simulink model "Clean_Tractor_Trailer_Flatness_v2"  (R2022b)
settings: Solver=ode4  StartTime=0.01  StopTime=20  FixedStep=0.01  RelTol=1e-3
InitFcn:
  | d0 = 1;
  | Dt=0.01;
  | 
  | %% if we want to "externalise" the trailer link from the car
  | a = 1.5;
  | 
  | %% distance between car and trailer
  | b = 2.5;
  | 
  | d1=b;
  | 
  | delay = 0.01;
  | 
  | %% delay with 0 signal before (to avoid instabilities before the "real" path following simulation")
  | del=2;
  | 
  | %% delay to sub above to chose starting using real value
  | dedel=1;
  | 
  | y0 = 0;
  | x0 = d1;
  | co=0;
  | 
  | the_pre=0;
  | the_pre_pre=0;
  | sdt=0.01;
  | 
  | ti_mod = 0.3;
  | 
  | phi0=pi;
  | 
  | %% Backward= pi, forward = 0
  | for_back=pi;
  | %%
  | 
  | %% Circle initial conditons forward
  | % for_back=0;
  | % dedel = 1.5;
  | % x_dot_init = 0;
  | % y_dot_init = 3;
  | % x_init = 0;
  | % y_init = 0;
  | % x0_init = b + del-dedel;
  | % y0_init = 0;
  | % theta0_init=for_back;
  | % theta1_init=0;
  | 
  | %% Circle initial conditons backward
  | % for_back=pi;
  | % dedel = 1.5;
  | % x_dot_init = 0;
  | % y_dot_init = 3;
  | % x_init = 0;
  | % y_init = 0;
  | % x0_init = -b;
  | % y0_init = 0;
  | % theta0_init=for_back;
  | % theta1_init=0;
  | 
  | %% func1 initial conditons
  | % x_dot_init = 1;
  | % y_dot_init = 0;
  | % x_init = 0;
  | % y_init = 0;
  | % x0_init = 0;
  | % y0_init = 0;
  | % theta0_init=0;
  | % theta1_init=0;
  | 
  | %% Wavy_up initial conditons
  | % x_dot_init = 0;
  | % y_dot_init = 0;
  | % x_init = 0;
  | % y_init = 0;
  | % x0_init = 0;
  | % y0_init = 0;
  | % theta0_init=0;
  | % theta1_init=0;
  | 
  | %% Backward Initial conditons for waving upward
  | for_back=pi;
  | x_dot_init = 1;
  | y_dot_init = 0;
  | 
  | x_init = 0;
  | y_init = 0;
  | 
  | %plant init
  | x0_init = -b;
  | y0_init = 0;
  | theta0_init=for_back;
  | theta1_init=0;
  | del=pi;
  | 
  | %% Forward Initial conditons for waving upward
  | % for_back=0;
  | % x_dot_init = 1;
  | % y_dot_init = 0;
  | %
  | % x_init = 0;
  | % y_init = 0;
  | %
  | % %plant init
  | % x0_init = b;
  | % y0_init = 0;
  | % theta0_init=for_back;
  | % theta1_init=0;
  | % del=pi;
  | 
  | 
  | %% Forward initial conditons for exp
  | % dedel=del;
  | % for_back=0;
  | % x_dot_init = 1;
  | % y_dot_init = 0;
  | % x_init = 0;
  | % y_init = 0;
  | % x0_init = 0;
  | % y0_init = 0;
  | % theta0_init=for_back;
  | % theta1_init=0;
  | 
  | %% Backward initial conditons for exp
  | % dedel=del-0.2;
  | % for_back=pi;
  | % x_dot_init = 1;
  | % y_dot_init = 0;
  | % x_init = 0;
  | % y_init = 0;
  | % x0_init = -b;
  | % y0_init = 0;
  | % theta0_init=for_back;
  | % theta1_init=0;
  | 
  | 
  | %% Cosinus initial conditons forward
  | % for_back=0;
  | % dedel=1;
  | % x_dot_init = 3;
  | % y_dot_init = 0;
  | % x_init = 0;
  | % y_init = 0;
  | % x0_init = b;
  | % y0_init = 0;
  | % theta0_init=for_back;
  | % theta1_init=0;
  | 
  | %% Cosinus initial conditons backward
  | % for_back=pi;
  | % dedel=1;
  | % x_dot_init = 3;
  | % y_dot_init = 0;
  | % x_init = 0;
  | % y_init = 0;
  | % x0_init = -b;
  | % y0_init = 0;
  | % theta0_init=for_back;
  | % theta1_init=0;
settings Model: Creator=chaudhuri  LastModifiedBy=Tugdual
settings ModelReferenceCC: EnableRefExpFcnMdlSchedulingChecks=on

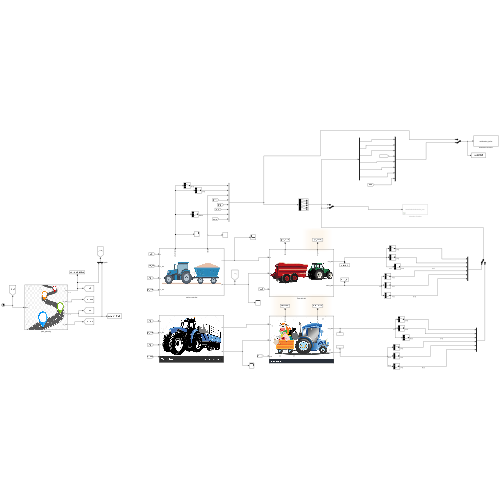
[thumbnail: Simulink's stored preview of the top-level diagram]
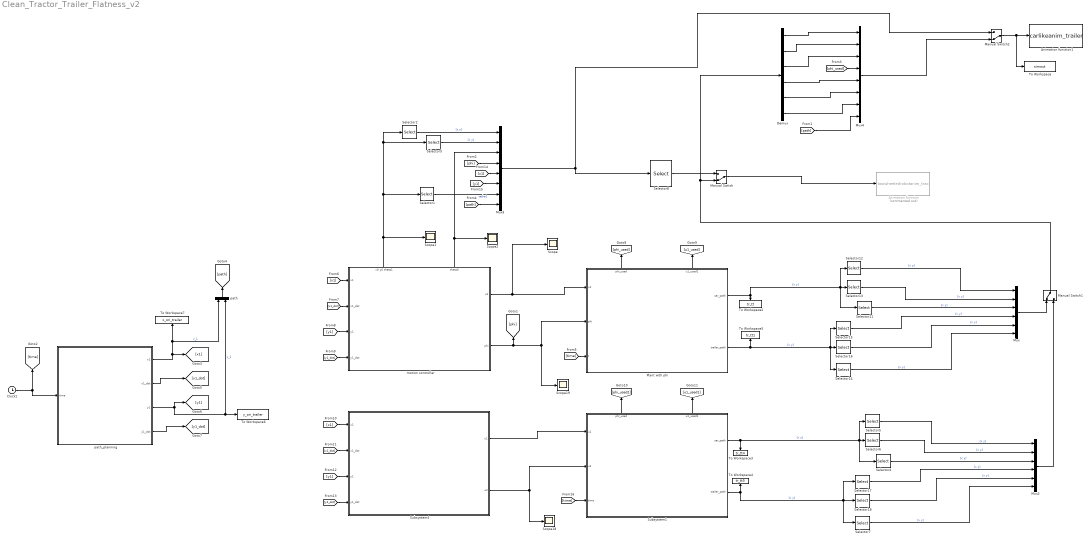
== system Clean_Tractor_Trailer_Flatness_v2 ==
  Animation function : S-Function  Commented=on  FunctionName=twowheeledrobotanim_trac  SFunctionDeploymentMode=off  EnableBusSupport=off
  Animation function1 : S-Function  FunctionName=carlikeanim_trailer  SFunctionDeploymentMode=off  EnableBusSupport=off
  Clock1 : Clock
  Demux : Demux  Outputs=6
  Manual Switch : ManualSwitch  CurrentSetting=0
  Manual Switch1 : ManualSwitch
  Manual Switch2 : ManualSwitch  CurrentSetting=0
  Mux : Mux  Inputs=6
  Mux2 : Mux  Inputs=6
  Mux3 : Mux  Inputs=8
  Mux4 : Mux  Inputs=8
  Plant with phi : Subsystem
      settings: PortSchema="{\"entries\":[{\"content\":{\"sides\":[{\"content\":{\"connectorIds\":[\"In1\",\"In2\",\"In3\"]},\"type\":\"ConnectorPlacement.EquallySpacedRectSide\",\"uuid\":\"e7db4861-1c7b-44d0-8ae0-043891a2d65e\"},{\"content\":{\"connectorIds\":[\"Out1\",\"Out2\"],\"side\":\"RIGHT\"},\"type\":\"ConnectorPlacement.EquallySpacedRectSide\",\"uuid\":\"ca6953ca-f3e9-441a-9b66-bf77f2babfba\"},{\"content\":{\"connectorIds\":[\"Out3\",\"Out4\"],\"side\":\"TOP\"},\"type\":\"ConnectorPlacement.EquallySpacedRectSide\",\"uuid\":\"0653e744-f46f-49ca-b3b7-6a2721aef055\"}]},\"type\":\"ConnectorPlacement.EquallySpacedConnector\",\"uuid\":\"d05efadf-1bd4-4ab0-9eff-99e9b7844dfa\"}],\"packageUris\":[\"http://schema.mathworks.com/mf0/Connector/R2020b\"],\"version\":\"1.0\"}"
      mask Display: image('$imagefile'); % Use "Edit Image" on toolstrip to change.
  Scope{,1..2,18..19} (5 alike) : Scope
  Selector{1,4,7,11,14} (5 alike) : Selector  InputPortWidth=3  IndexOptions=Index vector (dialog)  Indices=[3]  OutputSizes=1
  Selector{2,5,12,15,17} (5 alike) : Selector  InputPortWidth=3  IndexOptions=Index vector (dialog)  Indices=[1]  OutputSizes=1
  Selector{3,6,13,16,18} (5 alike) : Selector  InputPortWidth=3  IndexOptions=Index vector (dialog)  Indices=[2]  OutputSizes=1
  Selector8 : Selector  InputPortWidth=9  IndexOptions=Index vector (dialog)  Indices=[1 2 3 5 6 7]  OutputSizes=1
  Subsystem1 : Subsystem
      settings: PortSchema="{\"entries\":[{\"content\":{\"sides\":[{\"content\":{\"connectorIds\":[\"In1\",\"In2\",\"In3\"]},\"type\":\"ConnectorPlacement.EquallySpacedRectSide\",\"uuid\":\"e7db4861-1c7b-44d0-8ae0-043891a2d65e\"},{\"content\":{\"connectorIds\":[\"Out1\",\"Out2\"],\"side\":\"RIGHT\"},\"type\":\"ConnectorPlacement.EquallySpacedRectSide\",\"uuid\":\"ca6953ca-f3e9-441a-9b66-bf77f2babfba\"},{\"content\":{\"connectorIds\":[\"Out3\",\"Out4\"],\"side\":\"TOP\"},\"type\":\"ConnectorPlacement.EquallySpacedRectSide\",\"uuid\":\"0653e744-f46f-49ca-b3b7-6a2721aef055\"}]},\"type\":\"ConnectorPlacement.EquallySpacedConnector\",\"uuid\":\"d05efadf-1bd4-4ab0-9eff-99e9b7844dfa\"}],\"packageUris\":[\"http://schema.mathworks.com/mf0/Connector/R2020b\"],\"version\":\"1.0\"}"
      mask Display: image('$imagefile'); % Use "Edit Image" on toolstrip to change.
  Subsystem4 : Subsystem
      mask Display: image('$imagefile'); % Use "Edit Image" on toolstrip to change.
  To Workspace : ToWorkspace  VariableName=simout  SaveFormat=Timeseries  SampleTime=-1
  To Workspace2 : ToWorkspace  VariableName=tr_tt  SaveFormat=Timeseries  SampleTime=-1
  To Workspace3 : ToWorkspace  VariableName=tr_tt4  SaveFormat=Timeseries  SampleTime=-1
  To Workspace4 : ToWorkspace  VariableName=tr_tt5  SaveFormat=Timeseries  SampleTime=-1
  To Workspace5 : ToWorkspace  VariableName=tr_tt1  SaveFormat=Timeseries  SampleTime=-1
  To Workspace6 : ToWorkspace  VariableName=y_ori_trailer  SaveFormat=Timeseries  SampleTime=-1
      settings: Save2DSignal=2-D array (concatenate along first dimension)
  To Workspace7 : ToWorkspace  VariableName=x_ori_trailer  SaveFormat=Timeseries  SampleTime=-1
      settings: Save2DSignal=2-D array (concatenate along first dimension)
  motion controller : Subsystem
      settings: PortSchema="{\"entries\":[{\"content\":{\"sides\":[{\"content\":{\"connectorIds\":[\"In1\",\"In2\",\"In3\",\"In4\"]},\"type\":\"ConnectorPlacement.EquallySpacedRectSide\",\"uuid\":\"11bc3301-7ab6-4d38-8445-7de1e6050525\"},{\"content\":{\"connectorIds\":[\"Out1\",\"Out2\"],\"side\":\"RIGHT\"},\"type\":\"ConnectorPlacement.EquallySpacedRectSide\",\"uuid\":\"374bee85-8743-45f2-a60a-268bfdaad2ec\"},{\"content\":{\"connectorIds\":[\"Out3\",\"Out4\"],\"side\":\"TOP\"},\"type\":\"ConnectorPlacement.EquallySpacedRectSide\",\"uuid\":\"71c6a0a5-27e8-424b-8871-57b58ecd48a6\"}]},\"type\":\"ConnectorPlacement.EquallySpacedConnector\",\"uuid\":\"fb4e8639-9b4e-4508-bb82-15087a60f723\"}],\"packageUris\":[\"http://schema.mathworks.com/mf0/Connector/R2020b\"],\"version\":\"1.0\"}"
      mask Display: image('$imagefile'); % Use "Edit Image" on toolstrip to change.
  path : Mux  Inputs=2
  path_planning : Subsystem
      mask Display: image('$imagefile'); % Use "Edit Image" on toolstrip to change.
  wires:
  Subsystem4/1(u1) -> Subsystem1/1(u1)
  Subsystem4/2(u2) -> Scope18/1, Subsystem1/2(u2)
  Clock1/1 -> [time], path_planning/1(time)
  motion controller/2(phi) -> [phi], Plant with phi/2(phi), Scope19/1
  Plant with phi/1(car_path) -> Selector11/1, Selector12/1, Selector13/1, To Workspace2/1  "[x y]"
  Selector11/1 -> Mux/3  "[x y]"
  Selector12/1 -> Mux/1  "[x y]"
  Selector13/1 -> Mux/2  "[x y]"
  Selector16/1 -> Mux/5  "[x y]"
  Selector15/1 -> Mux/4  "[x y]"
  Plant with phi/2(trailer_path) -> Selector14/1, Selector15/1, Selector16/1, To Workspace5/1  "[x y]"
  Selector14/1 -> Mux/6  "[x y]"
  Manual Switch1/1 -> Demux/1, Manual Switch/2
  motion controller/1(u1) -> Plant with phi/1(u1), Scope/1
  motion controller/3(x0 y0 theta1) -> Scope1/1, Selector2/1, Selector3/1, Selector1/1
  Selector1/1 -> Mux3/7  "tetha1"
  Selector3/1 -> Mux3/2  "[x y]"
  Selector2/1 -> Mux3/1  "[x y]"
  Selector17/1 -> Mux2/4  "[x y]"
  Selector7/1 -> Mux2/6  "[x y]"
  Subsystem1/2(trailer_path) -> Selector7/1, Selector18/1, Selector17/1, To Workspace4/1  "[x y]"
  Selector18/1 -> Mux2/5  "[x y]"
  Subsystem1/1(car_path) -> Selector4/1, Selector5/1, Selector6/1, To Workspace3/1  "[x y]"
  Selector6/1 -> Mux2/2  "[x y]"
  Selector5/1 -> Mux2/1  "[x y]"
  Mux2/1 -> Manual Switch1/2
  Selector4/1 -> Mux2/3  "[x y]"
  Mux/1 -> Manual Switch1/1
  Manual Switch2/1 -> To Workspace/1, Animation function1/1
  Manual Switch/1 -> Animation function/1
  motion controller/4(theta0) -> Scope2/1, Mux3/3
  Mux4/1 -> Manual Switch2/2
  Mux3/1 -> Selector8/1, Manual Switch2/1
  Demux/1 -> Mux4/1
  Demux/2 -> Mux4/2
  Demux/3 -> Mux4/3
  Demux/4 -> Mux4/5
  Demux/5 -> Mux4/6
  Demux/6 -> Mux4/7
  path/1 -> [path]
  [path] -> Mux4/8
  [phi] -> Mux3/4
  [phi_used] -> Mux4/4
  [path] -> Mux3/8
  [time] -> Plant with phi/3(t)
  Selector8/1 -> Manual Switch/1
  [x1] -> Mux3/5
  [y1] -> Mux3/6
  [x1] -> motion controller/1(x1)
  [x1_dot] -> motion controller/2(x1_dot)
  [y1] -> motion controller/3(y1)
  [y1_dot] -> motion controller/4(y1_dot)
  [y1_dot] -> Subsystem4/4(y1_dot)
  [y1] -> Subsystem4/3(y1)
  [x1_dot] -> Subsystem4/2(x1_dot)
  [x1] -> Subsystem4/1(x1)
  path_planning/4(y1_dot) -> [y1_dot]
  path_planning/3(y1) -> [y1], To Workspace6/1, path/2  "y_1"
  path_planning/2(x1_dot) -> [x1_dot]
  path_planning/1(x1) -> path/1, To Workspace7/1, [x1]  "x_1"
  Plant with phi/3(phi_used) -> [phi_used]
  Plant with phi/4(u1_used1) -> [u1_used]
  [time] -> Subsystem1/3(time)
  Subsystem1/4(u1_used1) -> [u1_used1]
  Subsystem1/3(phi_used) -> [phi_used2]

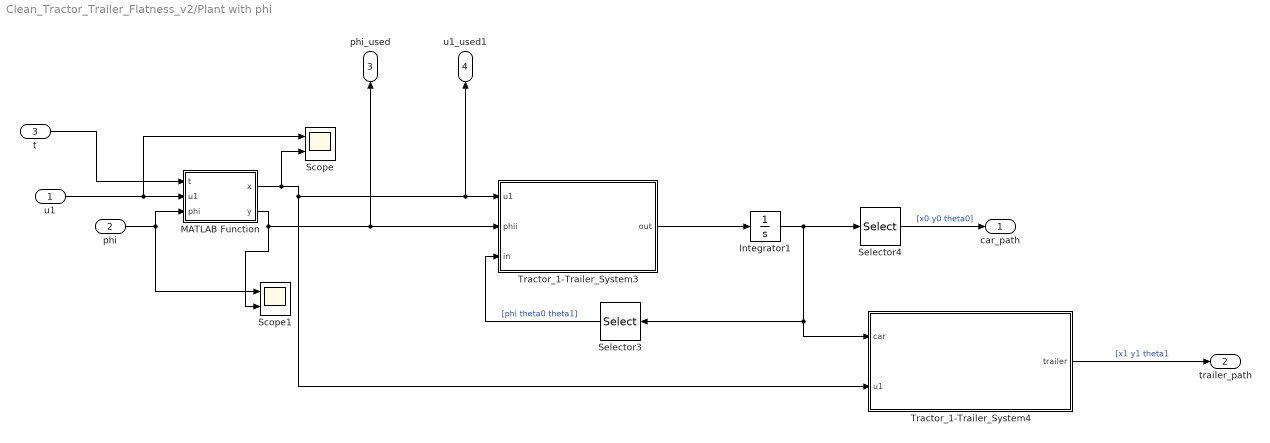
== system Clean_Tractor_Trailer_Flatness_v2/Plant with phi ==
  u1 : Inport
  phi : Inport  Port=2
  t : Inport  Port=3
  Integrator1 : Integrator  InitialCondition=[x0_init;y0_init;theta0_init;theta1_init]
  MATLAB Function : MATLAB Function  TreatAsAtomicUnit=on
  Scope : Scope  NumInputPorts=2
  Scope1 : Scope  NumInputPorts=2
  Selector3 : Selector  InputPortWidth=4  IndexOptions=Index vector (dialog)  Indices=[3 4]  OutputSizes=1
  Selector4 : Selector  InputPortWidth=4  IndexOptions=Index vector (dialog)  Indices=[1 2 3]  OutputSizes=1
  Tractor_1-Trailer_System3 : MATLAB Function  TreatAsAtomicUnit=on
  Tractor_1-Trailer_System4 : MATLAB Function  TreatAsAtomicUnit=on
  car_path : Outport
  trailer_path : Outport  Port=2
  phi_used : Outport  Port=3
  u1_used1 : Outport  Port=4
  wires:
  Tractor_1-Trailer_System4/1(trailer) -> trailer_path/1  "[x1 y1 theta1"
  Tractor_1-Trailer_System3/1(out) -> Integrator1/1
  Integrator1/1 -> Selector4/1, Tractor_1-Trailer_System4/1(car), Selector3/1
  Selector3/1 -> Tractor_1-Trailer_System3/3(in)  "[phi theta0 theta1]"
  Selector4/1 -> car_path/1  "[x0 y0 theta0]"
  MATLAB Function/2(y) -> Scope1/2, Tractor_1-Trailer_System3/2(phii), phi_used/1
  MATLAB Function/1(x) -> Scope/2, u1_used1/1, Tractor_1-Trailer_System3/1(u1), Tractor_1-Trailer_System4/2(u1)
  t/1 -> MATLAB Function/1(t)
  u1/1 -> Scope/1, MATLAB Function/2(u1)
  phi/1 -> Scope1/1, MATLAB Function/3(phi)

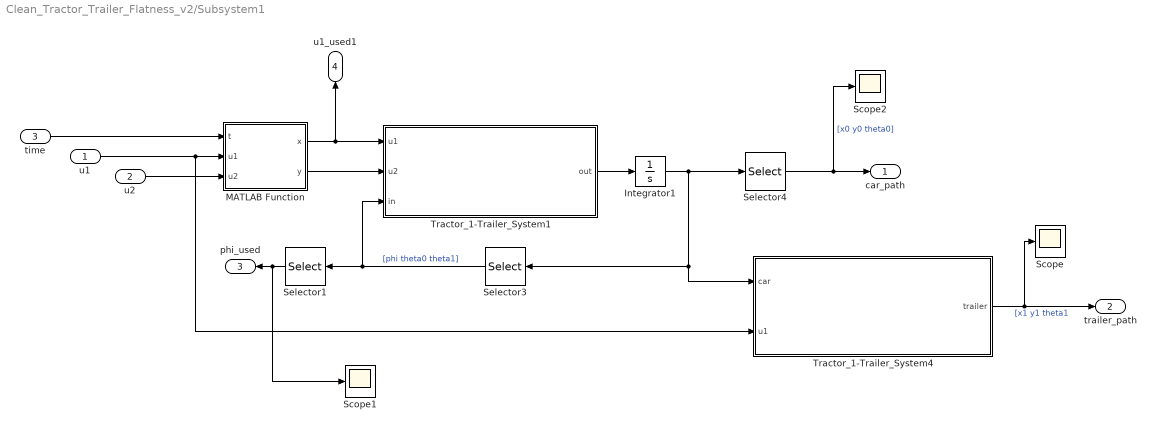
== system Clean_Tractor_Trailer_Flatness_v2/Subsystem1 ==
  u1 : Inport
  u2 : Inport  Port=2
  time : Inport  Port=3
  Integrator1 : Integrator  InitialCondition=[x0_init;y0_init;phi0;theta0_init;theta1_init]
  MATLAB Function : MATLAB Function  TreatAsAtomicUnit=on
  Scope : Scope
  Scope1 : Scope
  Scope2 : Scope
  Selector1 : Selector  InputPortWidth=3  IndexOptions=Index vector (dialog)  Indices=[1]  OutputSizes=1
  Selector3 : Selector  InputPortWidth=5  IndexOptions=Index vector (dialog)  Indices=[3 4 5]  OutputSizes=1
  Selector4 : Selector  InputPortWidth=5  IndexOptions=Index vector (dialog)  Indices=[1 2 4]  OutputSizes=1
  Tractor_1-Trailer_System1 : MATLAB Function  TreatAsAtomicUnit=on
  Tractor_1-Trailer_System4 : MATLAB Function  TreatAsAtomicUnit=on
  car_path : Outport
  trailer_path : Outport  Port=2
  phi_used : Outport  Port=3
  u1_used1 : Outport  Port=4
  wires:
  Tractor_1-Trailer_System4/1(trailer) -> Scope/1, trailer_path/1  "[x1 y1 theta1"
  Tractor_1-Trailer_System1/1(out) -> Integrator1/1
  Integrator1/1 -> Selector4/1, Tractor_1-Trailer_System4/1(car), Selector3/1
  Selector3/1 -> Selector1/1, Tractor_1-Trailer_System1/3(in)  "[phi theta0 theta1]"
  Selector4/1 -> Scope2/1, car_path/1  "[x0 y0 theta0]"
  u1/1 -> MATLAB Function/2(u1), Tractor_1-Trailer_System4/2(u1)
  u2/1 -> MATLAB Function/3(u2)
  time/1 -> MATLAB Function/1(t)
  MATLAB Function/1(x) -> u1_used1/1, Tractor_1-Trailer_System1/1(u1)
  MATLAB Function/2(y) -> Tractor_1-Trailer_System1/2(u2)
  Selector1/1 -> Scope1/1, phi_used/1

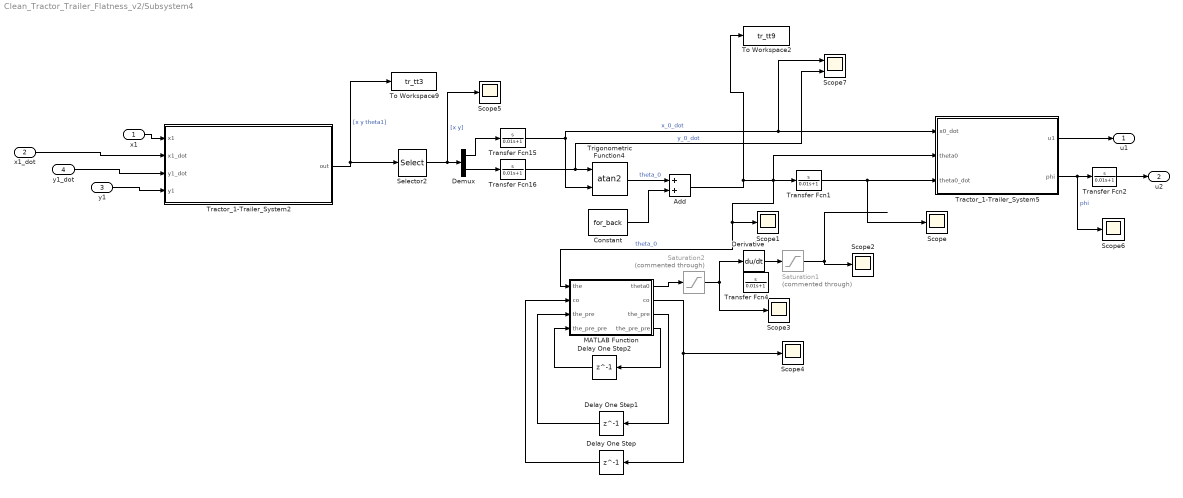
== system Clean_Tractor_Trailer_Flatness_v2/Subsystem4 ==
  x1 : Inport
  x1_dot : Inport  Port=2
  y1 : Inport  Port=3
  y1_dot : Inport  Port=4
  Add : Sum
  Constant : Constant  Value=for_back
  Delay One Step : Delay  DelayLength=1
  Delay One Step1 : Delay  DelayLength=1
  Delay One Step2 : Delay  DelayLength=1
  Demux : Demux  Outputs=2
  Derivative : Derivative
  MATLAB Function : MATLAB Function  TreatAsAtomicUnit=on
  Saturation1 : Saturate  Commented=through  UpperLimit=pi/4  LowerLimit=-pi/4
  Saturation2 : Saturate  Commented=through  UpperLimit=pi  LowerLimit=-pi
  Scope{,1..6} (7 alike) : Scope
  Scope7 : Scope  NumInputPorts=2
  Selector2 : Selector  InputPortWidth=3  IndexOptions=Index vector (dialog)  Indices=[1 2]  OutputSizes=1
  To Workspace2 : ToWorkspace  VariableName=tr_tt9  SaveFormat=Timeseries  SampleTime=-1
  To Workspace9 : ToWorkspace  VariableName=tr_tt3  SaveFormat=Timeseries  SampleTime=-1
  Tractor_1-Trailer_System2 : MATLAB Function  TreatAsAtomicUnit=on
  Tractor_1-Trailer_System5 : MATLAB Function  TreatAsAtomicUnit=on
  Transfer Fcn{1..2,4,15..16} (5 alike) : TransferFcn  Numerator=[1 0]  Denominator=[0.01 1]
  Trigonometric Function4 : Trigonometry  Operator=atan2
  u1 : Outport
  u2 : Outport  Port=2
  wires:
  Selector2/1 -> Scope5/1, Demux/1  "[x y]"
  Tractor_1-Trailer_System2/1(out) -> To Workspace9/1, Selector2/1  "[x y theta1]"
  Transfer Fcn16/1 -> Scope7/2, Trigonometric Function4/1  "y_0_dot"
  Transfer Fcn1/1 -> Scope/1, Tractor_1-Trailer_System5/3(theta0_dot)
  Transfer Fcn15/1 -> Trigonometric Function4/2, Scope7/1, Tractor_1-Trailer_System5/1(x0_dot)  "x_0_dot"
  Demux/2 -> Transfer Fcn16/1
  Demux/1 -> Transfer Fcn15/1
  Tractor_1-Trailer_System5/2(phi) -> Scope6/1, Transfer Fcn2/1  "phi"
  Tractor_1-Trailer_System5/1(u1) -> u1/1
  x1_dot/1 -> Tractor_1-Trailer_System2/2(x1_dot)
  Delay One Step/1 -> MATLAB Function/2("co ")
  MATLAB Function/1(theta0) -> Saturation2/1
  Add/1 -> To Workspace2/1, MATLAB Function/1(the), Scope1/1, Transfer Fcn1/1, Tractor_1-Trailer_System5/2(theta0)  "theta_0"
  MATLAB Function/2(co) -> Delay One Step/1, Scope4/1
  Derivative/1 -> Saturation1/1
  y1_dot/1 -> Tractor_1-Trailer_System2/3(y1_dot)
  y1/1 -> Tractor_1-Trailer_System2/4(y1)
  x1/1 -> Tractor_1-Trailer_System2/1(x1)
  Transfer Fcn2/1 -> u2/1
  Saturation1/1 -> Scope2/1
  Saturation2/1 -> Derivative/1, Scope3/1
  MATLAB Function/3(the_pre) -> Delay One Step1/1
  Delay One Step1/1 -> MATLAB Function/3("the_pre ")
  MATLAB Function/4(the_pre_pre) -> Delay One Step2/1
  Constant/1 -> Add/2
  Trigonometric Function4/1 -> Add/1  "theta_0"
  Delay One Step2/1 -> MATLAB Function/4("the_pre_pre ")

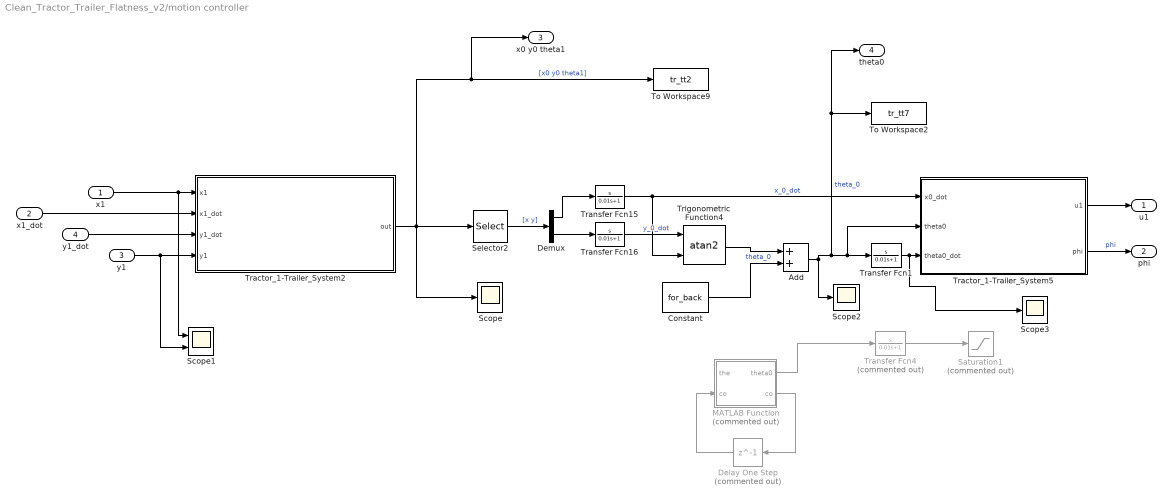
== system Clean_Tractor_Trailer_Flatness_v2/motion controller ==
  x1 : Inport
  x1_dot : Inport  Port=2
  y1 : Inport  Port=3
  y1_dot : Inport  Port=4
  Add : Sum
  Constant : Constant  Value=for_back
  Delay One Step : Delay  Commented=on  DelayLength=1
  Demux : Demux  Outputs=2
  MATLAB Function : MATLAB Function  Commented=on  TreatAsAtomicUnit=on
  Saturation1 : Saturate  Commented=on  UpperLimit=pi/4  LowerLimit=-pi/4
  Scope : Scope
  Scope1 : Scope  NumInputPorts=2
  Scope2 : Scope
  Scope3 : Scope
  Selector2 : Selector  InputPortWidth=3  IndexOptions=Index vector (dialog)  Indices=[1 2]  OutputSizes=1
  To Workspace2 : ToWorkspace  VariableName=tr_tt7  SaveFormat=Timeseries  SampleTime=-1
  To Workspace9 : ToWorkspace  VariableName=tr_tt2  SaveFormat=Timeseries  SampleTime=-1
  Tractor_1-Trailer_System2 : MATLAB Function  TreatAsAtomicUnit=on
  Tractor_1-Trailer_System5 : MATLAB Function  TreatAsAtomicUnit=on
  Transfer Fcn1 : TransferFcn  Numerator=[1 0]  Denominator=[0.01 1]
  Transfer Fcn15 : TransferFcn  Numerator=[1 0]  Denominator=[0.01 1]
  Transfer Fcn16 : TransferFcn  Numerator=[1 0]  Denominator=[0.01 1]
  Transfer Fcn4 : TransferFcn  Commented=on  Numerator=[1 0]  Denominator=[0.01 1]
  Trigonometric Function4 : Trigonometry  Operator=atan2
  u1 : Outport
  phi : Outport  Port=2
  x0 y0 theta1 : Outport  Port=3
  theta0 : Outport  Port=4
  wires:
  Selector2/1 -> Demux/1  "[x y]"
  Tractor_1-Trailer_System2/1(out) -> Scope/1, x0 y0 theta1/1, To Workspace9/1, Selector2/1  "[x0 y0 theta1]"
  Transfer Fcn16/1 -> Trigonometric Function4/1  "y_0_dot"
  Transfer Fcn1/1 -> Scope3/1, Tractor_1-Trailer_System5/3(theta0_dot)
  Add/1 -> theta0/1, To Workspace2/1, Tractor_1-Trailer_System5/2(theta0), Transfer Fcn1/1, Scope2/1  "theta_0"
  Transfer Fcn15/1 -> Tractor_1-Trailer_System5/1(x0_dot), Trigonometric Function4/2  "x_0_dot"
  Demux/2 -> Transfer Fcn16/1
  Demux/1 -> Transfer Fcn15/1
  Tractor_1-Trailer_System5/2(phi) -> phi/1  "phi"
  Tractor_1-Trailer_System5/1(u1) -> u1/1
  x1_dot/1 -> Tractor_1-Trailer_System2/2(x1_dot)
  Delay One Step/1 -> MATLAB Function/2("co ")
  MATLAB Function/1(theta0) -> Transfer Fcn4/1
  ? -> MATLAB Function/1(the)  "theta_0"
  MATLAB Function/2(co) -> Delay One Step/1
  Transfer Fcn4/1 -> Saturation1/1
  y1_dot/1 -> Tractor_1-Trailer_System2/3(y1_dot)
  y1/1 -> Scope1/2, Tractor_1-Trailer_System2/4(y1)
  x1/1 -> Scope1/1, Tractor_1-Trailer_System2/1(x1)
  Trigonometric Function4/1 -> Add/1  "theta_0"
  Constant/1 -> Add/2

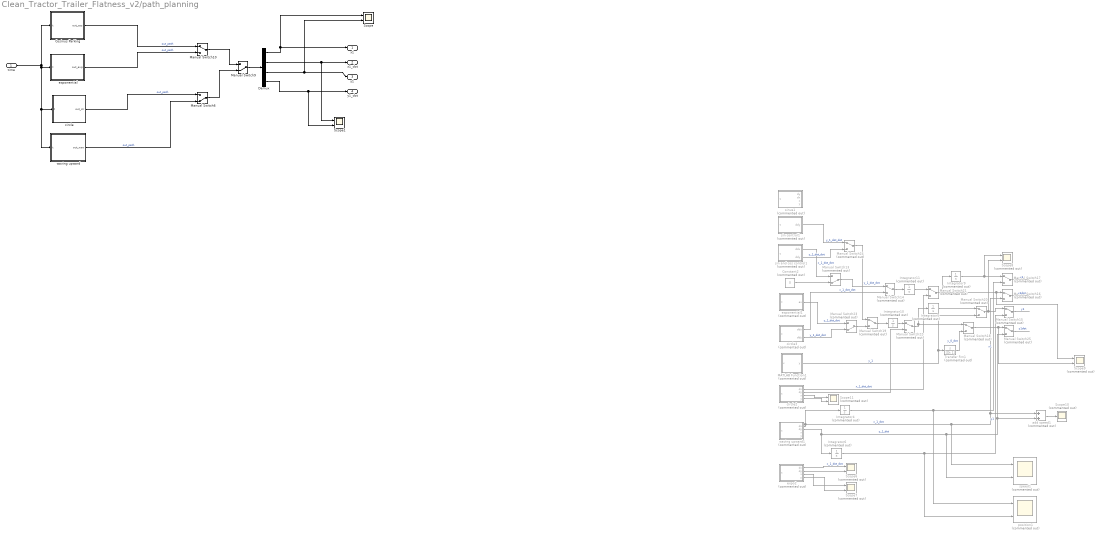
== system Clean_Tractor_Trailer_Flatness_v2/path_planning ==
  time : Inport
  Constant2 : Constant  Commented=on  Value=0
  Cosinus Parking : MATLAB Function  TreatAsAtomicUnit=on
  Demux : Demux
  Integrator10 : Integrator  Commented=on  InitialCondition=y_dot_init
  Integrator11 : Integrator  Commented=on  InitialCondition=x_dot_init
  Integrator4 : Integrator  Commented=on
  Integrator5 : Integrator  Commented=on  InitialCondition=y_init
  Integrator6 : Integrator  Commented=on
  Integrator9 : Integrator  Commented=on  InitialCondition=x_init
  MATLAB Function1 : MATLAB Function  Commented=on  TreatAsAtomicUnit=on
  Manual Switch10 : ManualSwitch
  Manual Switch13 : ManualSwitch  Commented=on  CurrentSetting=0
  Manual Switch{14..22,24..25} (11 alike) : ManualSwitch  Commented=on
  Manual Switch23 : ManualSwitch  Commented=on  CurrentSetting=0
  Manual Switch6 : ManualSwitch  CurrentSetting=0
  Manual Switch9 : ManualSwitch  CurrentSetting=0
  Scope : Scope  NumInputPorts=2
  Scope1 : Scope  NumInputPorts=2
  Scope10 : Scope  Commented=on
  Scope{6..9,11} (5 alike) : Scope  Commented=on  NumInputPorts=2
  Transfer Fcn1 : TransferFcn  Commented=on  Numerator=[1 0]  Denominator=[Dt 1]
  add speed1 : Sum  Commented=on
  circle : MATLAB Function  TreatAsAtomicUnit=on
  circle2 : MATLAB Function  Commented=on  TreatAsAtomicUnit=on
  circle3 : MATLAB Function  Commented=on  TreatAsAtomicUnit=on
  expo2 : MATLAB Function  Commented=on  TreatAsAtomicUnit=on
  exponential : MATLAB Function  TreatAsAtomicUnit=on
  exponential1 : MATLAB Function  Commented=on  TreatAsAtomicUnit=on
  position1 : Scope  Commented=on  NumInputPorts=2
  sin and cos control1 : MATLAB Function  Commented=on  TreatAsAtomicUnit=on
  sin control1 : MATLAB Function  Commented=on  TreatAsAtomicUnit=on
  sinus1 : MATLAB Function  Commented=on  TreatAsAtomicUnit=on
  speed1 : Scope  Commented=on  NumInputPorts=2
  waving upward : MATLAB Function  TreatAsAtomicUnit=on
  waving upward1 : MATLAB Function  Commented=on  TreatAsAtomicUnit=on
  x1 : Outport
  x1_dot : Outport  Port=2
  y1 : Outport  Port=3
  y1_dot : Outport  Port=4
  wires:
  exponential/1(out_exp) -> Manual Switch10/2  "out_path"
  time/1 -> exponential/1(t), waving upward/1(t), circle/1(t), Cosinus Parking/1(t)
  circle2/4(y) -> Scope11/2
  Manual Switch16/1 -> ?  "x1dot"
  Manual Switch15/1 -> ?  "y1"
  Manual Switch19/1 -> Integrator10/1
  expo2/3(x) -> Scope7/1
  circle2/2(dy) -> Manual Switch22/2
  circle3/2(ddy) -> Manual Switch23/2  "y_1_dot_dot"
  expo2/2(dy) -> Scope6/2
  Integrator6/1 -> position1/2, Manual Switch15/2  "y1"
  add speed1/1 -> Scope10/1
  waving upward1/2(dy) -> add speed1/2, Manual Switch25/2, speed1/2, Integrator6/1  "y_1_dot"
  Manual Switch21/1 -> Scope9/1, Manual Switch16/1, Integrator9/1
  Manual Switch18/1 -> Scope9/2, Manual Switch25/1
  Integrator5/1 -> Manual Switch20/1
  sin and cos control1/2(ddy) -> Manual Switch24/2  "y_1_dot_dot"
  Manual Switch17/1 -> ?  "x1"
  Integrator10/1 -> Manual Switch22/1
  expo2/4(y) -> Scope7/2
  Integrator9/1 -> Scope8/1, Manual Switch17/1
  circle2/1(dx) -> Manual Switch21/2  "x_1_dot_dot"
  waving upward1/1(dx) -> add speed1/1, Manual Switch16/2, speed1/1, Integrator4/1  "x_1_dot"
  Manual Switch14/1 -> Integrator11/1
  Integrator4/1 -> position1/1, Manual Switch17/2  "x1"
  Manual Switch25/1 -> ?  "y1dot"
  expo2/1(dx) -> Scope6/1  "x_1_dot_dot"
  ? -> exponential1/1(t), sin control1/1(t), sinus1/1(t), sin and cos control1/1(t), circle3/1(t), MATLAB Function1/1(x), expo2/1(t), waving upward1/1(t), circle2/1(t)
  Integrator11/1 -> Manual Switch21/1
  exponential1/1(ex) -> Manual Switch23/1  "y_1_dot_dot"
  sin and cos control1/1(ddx) -> Manual Switch13/1  "x_1_dot_dot"
  Manual Switch13/1 -> Manual Switch14/1
  MATLAB Function1/1(y) -> Manual Switch20/2, Transfer Fcn1/1  "y_1"
  circle3/1(ddx) -> Manual Switch14/2  "x_1_dot_dot"
  Manual Switch24/1 -> Manual Switch19/1  "y_1_dot_dot"
  Transfer Fcn1/1 -> Manual Switch18/2  "y_0_dot"
  Manual Switch22/1 -> Integrator5/1, Manual Switch18/1
  Manual Switch20/1 -> Scope8/2, Manual Switch15/1
  Constant2/1 -> Manual Switch13/2
  circle2/3(x) -> Scope11/1
  sin control1/1(ddy) -> Manual Switch24/1  "y_1_dot_dot"
  Manual Switch23/1 -> Manual Switch19/2
  Demux/1 -> x1/1, Scope/1
  Demux/2 -> Scope1/1, x1_dot/1
  Demux/3 -> y1/1, Scope/2
  Demux/4 -> Scope1/2, y1_dot/1
  Manual Switch9/1 -> Demux/1
  waving upward/1(out_wav) -> Manual Switch6/2  "out_path"
  Cosinus Parking/1(out_cos) -> Manual Switch10/1  "out_path"
  Manual Switch10/1 -> Manual Switch9/1
  circle/1(out_cir) -> Manual Switch6/1  "out_path"
  Manual Switch6/1 -> Manual Switch9/2

== matlab function Clean_Tractor_Trailer_Flatness_v2/motion controller/Tractor_1-Trailer_System2 ==
  data: x1 input; x1_dot input; out output; y1_dot input; y1 input; d1 parameter; for_back parameter
function out = fcn(x1,x1_dot, y1_dot, y1, d1,for_back)
%% Trying to approximate tangente function with Leonhard Euler and then taylor series 
% the11=0;
% for n = 0:100
%     if n==0
%         the11=1*(y1_dot/x1_dot)/(1+(y1_dot/x1_dot));
%     else
%         prod=1;
%         for k = 1:n
%             prod=2*k*((y1_dot/x1_dot)^2)/((2*k+1)*(1+(y1_dot/x1_dot)^2));
%         end
%         the11=the11+prod*(y1_dot/x1_dot)/(1+(y1_dot/x1_dot)^2);
%     end
% end
% the111=0;
% for n = 0:100
%     the111=the111+((-1)^n)*((y1_dot/x1_dot)^(2*n+1))/(2*n+1);
% end
% the111=the111-for_back;
% the11=the11-for_back;

theta1 = atan2(y1_dot,x1_dot)-for_back;
% theta1 = atan2(y1,x1)-for_back;
y0 = y1 + d1*sin(theta1);
x0 = x1 + d1*cos(theta1);

out=[x0;y0;theta1];

== matlab function Clean_Tractor_Trailer_Flatness_v2/Subsystem1/MATLAB Function ==
  data: t input; x output; u1 input; y output; u2 input; del parameter; dedel parameter
function [x,y]= fcn(t,u1,u2,del, dedel)
if t<del-dedel
    x=-2;
    y=0;
else
    x=u1;
    y=u2;
end

== matlab function Clean_Tractor_Trailer_Flatness_v2/path_planning/Cosinus Parking ==
  data: t input; out_cos output
function out_cos = fcn(t)
if t<pi | t > 3*pi 
    x=2*t;
    y=0;
    dx=2;
    dy=0;
else
    x=2*t;
    y=cos(t)-cos(pi);
    dx=2;
    dy=-sin(t);
end
out_cos=[x, dx, y, dy];

%% tring to fix the jumps
% function out_cos = fcn(t)
% if t<pi | t > 3*pi 
%     x=2*t;
%     y=0;
%     dy=0;
%     dx=2;
% else
%     y=cos(t)-cos(pi);
%     x=sqrt(4*t^2-y^2);
%     dy=-sin(t);
%     dx=sqrt(4-dy^2);
% end
% out_cos=[x, dx, y, dy];

== matlab function Clean_Tractor_Trailer_Flatness_v2/motion controller/Tractor_1-Trailer_System5 ==
  data: u1 output; x0_dot input; theta0 input; phi output; theta0_dot input; d0 parameter
function [u1, phi]= fcn(x0_dot, theta0, theta0_dot, d0)
u1 = x0_dot/(cos(theta0));
phi = atan2(d0*theta0_dot,u1);

== matlab function Clean_Tractor_Trailer_Flatness_v2/motion controller/MATLAB Function ==
  data: the input; theta0 output; co input; co output
function [theta0,co]= fcn(the,co)
if u < -pi+0.005
    co = co + 2*pi;
end
theta0 = the - co;

== matlab function Clean_Tractor_Trailer_Flatness_v2/path_planning/waving upward ==
  data: out_wav output; t input
function out_wav = fcn(t)
if t<pi
    
    dy=0;
    y=0;
    x=2*t;
    dx=sqrt(4-dy^2);
else
dy=cos(t)+1;

y=sin(t) + t-pi;
x=-sin(t)+t+pi;
dx=-(cos(t)+1)+2;
end
out_wav = [x,dx,y,dy];

== matlab function Clean_Tractor_Trailer_Flatness_v2/Subsystem4/MATLAB Function ==
  data: the input; theta0 output; co input; co output; the_pre input; the_pre output; the_pre_pre input; the_pre_pre output
function [theta0,co,the_pre,the_pre_pre]= fcn(the,co,the_pre,the_pre_pre)
%tempp=the_pre
if abs(the) > pi-0.01
    co = co + 2*pi*abs(the_pre)/the_pre;
end
% if abs(the) > pi-0.01 && the_pre - the > 0
%     co = co + 2*pi*abs(the_pre)/the_pre;
%     the_pre = pi;
% elseif the > pi-0.01 && the_pre - the < 0
%         co = co + 2*pi;
%         the_pre = -pi;
% else
%     the_pre = the;
% end

theta0 = the + co;

if abs(theta0 - the_pre) > 2 
    theta0 = the_pre + (the_pre-the_pre_pre);
end

the_pre_pre = the_pre;
the_pre = theta0;

== matlab function Clean_Tractor_Trailer_Flatness_v2/Subsystem4/Tractor_1-Trailer_System2 ==
  data: x1 input; x1_dot input; out output; y1_dot input; y1 input; d1 parameter; for_back parameter
function out = fcn(x1,x1_dot, y1_dot, y1, d1,for_back)
theta1 = atan2(y1_dot,x1_dot)+for_back;
y0 = y1 + d1*sin(theta1);
x0 = x1 + d1*cos(theta1);
out=[x0;y0;theta1];

== matlab function Clean_Tractor_Trailer_Flatness_v2/path_planning/exponential ==
  data: t input; out_exp output; ti_mod parameter; dedel parameter; del parameter
% function out_exp = fcn(t,ti_mod)
% if t<3
%     y=exp(t*ti_mod)-1;
% %     y=exp(t-6);
%     x=2*t;
%     dx=2;
%     dy=ti_mod*exp(t*ti_mod);
% %     dy=exp(t-6);
% else
% %     y=exp(ti_mod*t+3*(1-ti_mod)-2);
%     y=exp(t*ti_mod)-1;
%     x=2*t;
%     dx=2;
%     dy=ti_mod*exp(t*ti_mod);
% %     dy=ti_mod*exp(ti_mod*t-6);
% end
% out_exp=[x,dx,y,dy];

function out_exp = fcn(t,ti_mod,dedel, del)
if t<del-dedel
    y=0;
%     y=exp(t-6);
    x=2*t;
    dx=2;
    dy=0;
%     dy=exp(t-6);
else
%     y=exp(ti_mod*t+3*(1-ti_mod)-2);
    y=exp((t-dedel)*ti_mod)-1;
    x=2*t;
    dx=2;
    dy=ti_mod*exp((t-dedel)*ti_mod);
%     dy=ti_mod*exp(ti_mod*t-6);
end
out_exp=[x,dx,y,dy];

== matlab function Clean_Tractor_Trailer_Flatness_v2/Subsystem4/Tractor_1-Trailer_System5 ==
  data: u1 output; x0_dot input; theta0 input; phi output; theta0_dot input; d0 parameter
function [u1, phi]= fcn(x0_dot, theta0, theta0_dot, d0)
u1 = x0_dot/(cos(theta0));
phi = atan2(d0*theta0_dot,u1);

== matlab function Clean_Tractor_Trailer_Flatness_v2/path_planning/MATLAB Function1 ==
  data: x input; y output
function y = fcn(x)
y=100*(- (62962620750085869*x^8)/39614081257132168796771975168 + (575738832333271*x^7)/1208925819614629174706176 - (4389382977429541*x^6)/75557863725914323419136 + (8743933779681435*x^5)/2361183241434822606848 - (19457625648948835*x^4)/147573952589676412928 + (6015483242436685*x^3)/2305843009213693952 - (15450301083236355*x^2)/576460752303423488 + (277*x)/2500 + 4819/100000);

== matlab function Clean_Tractor_Trailer_Flatness_v2/path_planning/circle2 ==
  data: dx output; t input; dy output; x output; y output
function [dx,dy,x,y]= fcn(t)
if t<=1
    dx=3;
    x = 3*t;
    dy=0;
    y=0;
else
dy=-3*sin(t-1);
dx=3*cos(t-1);
x= 3 * sin(t-1) + 3;
y = 3*cos(t-1) - 3;
end

== matlab function Clean_Tractor_Trailer_Flatness_v2/path_planning/circle3 ==
  data: ddx output; t input; ddy output
function [ddx,ddy]= fcn(t)
ddy=-3*cos(t);
ddx=3*sin(t);

== matlab function Clean_Tractor_Trailer_Flatness_v2/path_planning/expo2 ==
  data: dx output; t input; dy output; x output; y output; del parameter
function [dx,dy,x,y]= fcn(t,del)
if t<del
    dx=2;
    dy=0;
    y=0;
    x=2*t;
else
dy=0.3*exp((t-2)*0.3)-0.3;
dx=2;
x=2*t;
y=exp((t-2)*0.3)-1;
end

== matlab function Clean_Tractor_Trailer_Flatness_v2/path_planning/exponential1 ==
  data: t input; ex output; ti_mod parameter
function ex = fcn(t,ti_mod)
if t<0
    ex=0
else
    ex=exp(ti_mod*t-0);
end

== matlab function Clean_Tractor_Trailer_Flatness_v2/path_planning/sin and cos control1 ==
  data: ddx output; t input; ddy output; ti_mod parameter
function [ddx,ddy]= fcn(t,ti_mod)
ddy=1.8*cos(ti_mod*t);
ddx=5*sin(t);

== matlab function Clean_Tractor_Trailer_Flatness_v2/path_planning/sin control1 ==
  data: t input; ddy output
function ddy = fcn(t)
if t<1
    ddy=0;
else
ddy=-2*cos(t);
end

== matlab function Clean_Tractor_Trailer_Flatness_v2/path_planning/sinus1 ==
  data: t input; dy output; dx output; x output; y output
function [dy, dx, x, y]= fcn(t)
if t<pi
    x=t;
    y=0;
    dx=1;
    dy=0;
else
    x=t;
    y=cos(t)-cos(pi);
    dx=1;
    dy=-sin(t);
end

== matlab function Clean_Tractor_Trailer_Flatness_v2/path_planning/waving upward1 ==
  data: dx output; t input; dy output; x output; y output
function [dx,dy,x,y]= fcn(t)
if t<pi
    
    dy=0;
    y=0;
    x=2*t;
    dx=sqrt(4-dy^2);
else
dy=cos(t)+1;

y=sin(t) + t-pi;
x=-sin(t)+t+pi;
dx=-(cos(t)+1)+2;
end

== matlab function Clean_Tractor_Trailer_Flatness_v2/Plant with phi/Tractor_1-Trailer_System3 ==
  data: out output; u1 input; phii input; in input; a parameter; b parameter; d0 parameter; d1 parameter
function out = fcn(u1, phii, in, a, b, d0, d1)

phi = phii;
theta0 = in(1);
theta1 = in(2);

x0_dot = cos(theta0)*u1;
y0_dot = sin(theta0)*u1;

theta0_dot = (1/d0)*tan(phi)*u1;
%theta1_dot = (1/b)*((a/d0)*tan(phi)*cos(theta0 - theta1) - sin(theta0 - theta1))*u1;
% theta1_dot = (1/d1)*cos(theta0 - theta1)*sin(theta0-theta1)*u1;
% theta1_dot = (1/d1)*((a/d0)*tan(phi)*cos(theta0 - theta1) - sin(theta0 - theta1))*u1;
theta1_dot = (1/d1)*(sin(theta0 - theta1))*u1*sign(u1);

out = [x0_dot;y0_dot;theta0_dot;theta1_dot];

== matlab function Clean_Tractor_Trailer_Flatness_v2/Plant with phi/Tractor_1-Trailer_System4 ==
  data: trailer output; car input; d1 parameter; u1 input; for_back parameter
function trailer= fcn(car,d1,u1,for_back)

trailer = [car(1) - sign(u1)*d1*cos(car(4));car(2) - sign(u1)*d1*sin(car(4));car(4)+for_back];

== matlab function Clean_Tractor_Trailer_Flatness_v2/Plant with phi/MATLAB Function ==
  data: t input; x output; u1 input; y output; phi input; del parameter; dedel parameter; for_back parameter
function [x,y]= fcn(t,u1,phi,del, dedel, for_back)
if t<del-dedel
    if for_back == 0
        x=2;
    else
        x=-2;
    end
    y=for_back;
else
    x=u1;
    y=phi;
end

== matlab function Clean_Tractor_Trailer_Flatness_v2/Subsystem1/Tractor_1-Trailer_System1 ==
  data: out output; u1 input; u2 input; in input; a parameter; b parameter; d0 parameter; d1 parameter
function out = fcn(u1, u2, in, a, b, d0, d1)

phi = in(1);
theta0 = in(2);
theta1 = in(3);

x0_dot = cos(theta0)*u1;
y0_dot = sin(theta0)*u1;
phi_dot = u2;

theta0_dot = (1/d0)*tan(phi)*u1;
%theta1_dot = (1/b)*((a/d0)*tan(phi)*cos(theta0 - theta1) - sin(theta0 - theta1))*u1;
% theta1_dot = (1/d1)*cos(theta0 - theta1)*sin(theta0-theta1)*u1;
% theta1_dot = (1/d1)*((a/d0)*tan(phi)*cos(theta0 - theta1) - sin(theta0 - theta1))*u1;
theta1_dot = (1/d1)*(sin(theta0 - theta1))*u1*sign(u1);

out = [x0_dot;y0_dot;phi_dot;theta0_dot;theta1_dot];

== matlab function Clean_Tractor_Trailer_Flatness_v2/path_planning/circle ==
  data: out_cir output; t input
function out_cir= fcn(t)
if t<=1
    dx=3;
    x = 3*t;
    dy=0;
    y=0;
else
dy=-3*sin(t-1);
dx=3*cos(t-1);
x= 3 * sin(t-1) + 3;
y = 3*cos(t-1) - 3;
end
out_cir=[x,dx,y,dy];

== matlab function Clean_Tractor_Trailer_Flatness_v2/Subsystem1/Tractor_1-Trailer_System4 ==
  data: trailer output; car input; d1 parameter; u1 input; for_back parameter
function trailer= fcn(car,d1,u1,for_back)

trailer = [car(1) - d1*cos(car(5))*sign(u1);car(2) - d1*sin(car(5))*sign(u1);car(5)+for_back];
